simulink model "Bldc"  (R2020a)
settings: Solver=VariableStepAuto  StartTime=0.0  StopTime=10.0  RelTol=1e-3
libraries: simulink x7
settings Model: Creator=kolep  LastModifiedBy=kolep

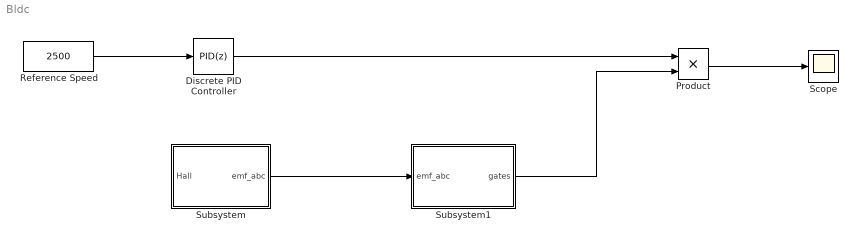
== system Bldc ==
  Discrete PID Controller : simulink/Continuous/PID Controller  Controller=PID  Form=Parallel  TimeDomain=Discrete-time  UseExternalTs=off  SampleTime=-1  IntegratorMethod=Forward Euler  FilterMethod=Forward Euler  ControllerParametersSource=internal  P=1  I=1  D=0  UseFilter=on  N=100  TunerSelectOption=Transfer Function Based (PID Tuner App)  InitialConditionSource=internal  InitialConditionForIntegrator=0  InitialConditionForFilter=0  DifferentiatorICPrevScaledInput=0  ExternalReset=none  TrackingMode=off  Kt=1  LimitOutput=off  UpperSaturationLimit=inf  LowerSaturationLimit=-inf  LinearizeAsGain=off  AntiWindupMode=none  Kb=1  POutMin=[]  POutMax=[]  IOutMin=[]  IOutMax=[]  DOutMin=[]  DOutMax=[]  NOutMin=[]  NOutMax=[]  SumOutMin=[]  SumOutMax=[]  SaturationOutMin=[]  SaturationOutMax=[]  PParamMin=[]  PParamMax=[]  IParamMin=[]  IParamMax=[]  DParamMin=[]  DParamMax=[]  NParamMin=[]  NParamMax=[]  KbParamMin=[]  KbParamMax=[]  KtParamMin=[]  KtParamMax=[]  KbOutMin=[]  KbOutMax=[]  KtOutMin=[]  KtOutMax=[]  IntegratorOutMin=[]  IntegratorOutMax=[]  FilterOutMin=[]  FilterOutMax=[]  SumI1OutMin=[]  SumI1OutMax=[]  SumI2OutMin=[]  SumI2OutMax=[]  SumI3OutMin=[]  SumI3OutMax=[]  SumI4OutMin=[]  SumI4OutMax=[]  SumDOutMin=[]  SumDOutMax=[]  DifferentiatorOutMin=[]  DifferentiatorOutMax=[]  FilterDiffOutCoefMin=[]  FilterDiffOutCoefMax=[]  ReciprocalOutMin=[]  ReciprocalOutMax=[]  SumDenOutMin=[]  SumDenOutMax=[]  SumNumOutMin=[]  SumNumOutMax=[]  DivideOutMin=[]  DivideOutMax=[]  UdiffTsProdOutMin=[]  UdiffTsProdOutMax=[]  NTsProdOutMin=[]  NTsProdOutMax=[]  UintegralTsProdOutMin=[]  UintegralTsProdOutMax=[]  UngainTsProdOutMin=[]  UngainTsProdOutMax=[]  IntegratorContinuousStateAttributes=''  IntegratorStateMustResolveToSignalObject=off  IntegratorRTWStateStorageClass=Auto  FilterContinuousStateAttributes=''  FilterStateMustResolveToSignalObject=off  FilterRTWStateStorageClass=Auto  ParallelPVariant=InternalParameters  IdealPVariant=Disabled  IVariant=InternalParameters  DVariant=InternalParameters  IntegratorVariant=Discrete  SatVariant=Disabled  AWVariant=Passthrough  PCopyVariant=Disabled  TRVariant=Disabled  FdbkBlocksVariant=Forward  IdealPFdbkVariant=Disabled  SatFdbkVariant=Disabled  DerivativeFilterVariant=ForwardEulerFilter  NVariant=InternalParameters  NCopyVariant=Disabled  FilterICVariant=InternalICsFilter  IntegratorICVariant=InternalICs  ExternalResetVariant=Disabled  TRSumVariant=Passthrough  SumFdbkVariant=Disabled  SumVariant=Sum_PID  TsampFilterVariant=InternalTs  TsampNgainVariant=Passthrough  TsampIntegralVariant=Passthrough
  Product : Product
  Reference Speed : Constant  Value=2500
  Scope : Scope
  Subsystem : Subsystem
  Subsystem1 : Subsystem
  wires:
  Reference Speed/1 -> Discrete PID Controller/1
  Discrete PID Controller/1 -> Product/1
  Subsystem/1(emf_abc) -> Subsystem1/1(emf_abc)
  Subsystem1/1(gates) -> Product/2
  Product/1 -> Scope/1

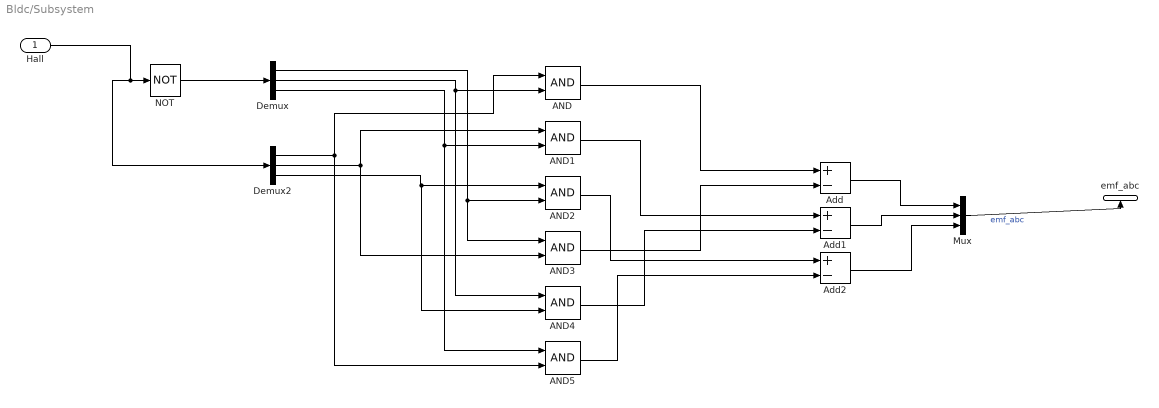
== system Bldc/Subsystem ==
  Hall : Inport
  AND{,1..5} (6 alike) : Logic  AllPortsSameDT=off  OutDataTypeStr=boolean
  Add : Sum  Inputs=+-
  Add1 : Sum  Inputs=+-
  Add2 : Sum  Inputs=+-
  Demux : Demux  Outputs=3
  Demux2 : Demux  Outputs=3
  Mux : Mux  Inputs=3
  NOT : Logic  Operator=NOT  AllPortsSameDT=off  OutDataTypeStr=boolean
  emf_abc : Outport
  wires:
  Hall/1 -> Demux2/1, NOT/1
  Demux2/3 -> AND4/2, AND2/1
  AND5/1 -> Add2/2
  NOT/1 -> Demux/1
  AND4/1 -> Add1/2
  Demux/3 -> AND5/1, AND1/2
  AND1/1 -> Add1/1
  AND2/1 -> Add2/1
  Demux2/1 -> AND/1, AND5/2
  Demux2/2 -> AND1/1, AND3/2
  AND/1 -> Add/1
  Demux/2 -> AND4/1, AND/2
  Demux/1 -> AND2/2, AND3/1
  Add1/1 -> Mux/2
  Add2/1 -> Mux/3
  Add/1 -> Mux/1
  AND3/1 -> Add/2
  Mux/1 -> emf_abc/1  "emf_abc"

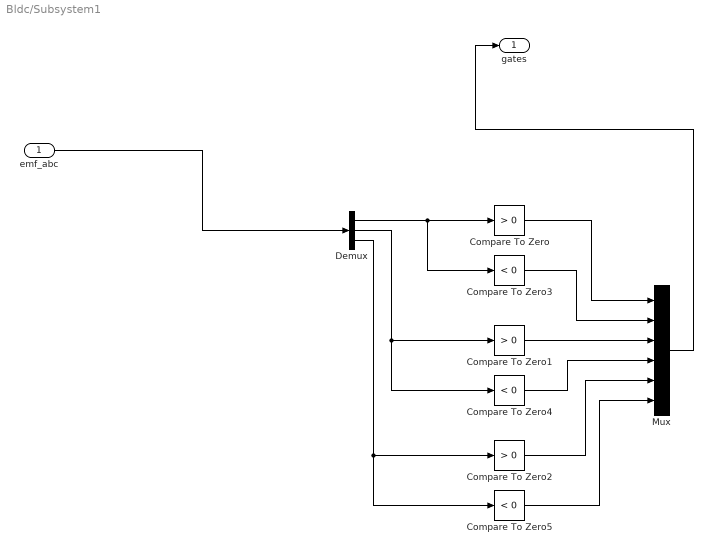
== system Bldc/Subsystem1 ==
  emf_abc : Inport
  Compare To Zero : simulink/Logic and Bit Operations/Compare To Zero  relop=>  OutDataTypeStr=boolean
  Compare To Zero1 : simulink/Logic and Bit Operations/Compare To Zero  relop=>  OutDataTypeStr=boolean
  Compare To Zero2 : simulink/Logic and Bit Operations/Compare To Zero  relop=>  OutDataTypeStr=boolean
  Compare To Zero3 : simulink/Logic and Bit Operations/Compare To Zero  relop=<  OutDataTypeStr=boolean
  Compare To Zero4 : simulink/Logic and Bit Operations/Compare To Zero  relop=<  OutDataTypeStr=boolean
  Compare To Zero5 : simulink/Logic and Bit Operations/Compare To Zero  relop=<  OutDataTypeStr=boolean
  Demux : Demux  Outputs=3
  Mux : Mux  Inputs=6
  gates : Outport
  wires:
  Compare To Zero5/1 -> Mux/6
  Compare To Zero/1 -> Mux/1
  Demux/2 -> Compare To Zero4/1, Compare To Zero1/1
  Compare To Zero3/1 -> Mux/2
  Demux/1 -> Compare To Zero3/1, Compare To Zero/1
  Demux/3 -> Compare To Zero5/1, Compare To Zero2/1
  Compare To Zero1/1 -> Mux/3
  Compare To Zero4/1 -> Mux/4
  emf_abc/1 -> Demux/1
  Compare To Zero2/1 -> Mux/5
  Mux/1 -> gates/1
